simulink model "Dc_motor_pi_camp_quant"  (R2021b)
settings: Solver=VariableStepAuto  StartTime=0.0  StopTime=10.0  RelTol=1e-3
InitFcn:
  | sampling=0.01;
  | quant_err=0.0001;
settings Model: Creator=Omar  LastModifiedBy=Omar
settings DebuggingCC: UnderSpecifiedDimensionMsg=warning

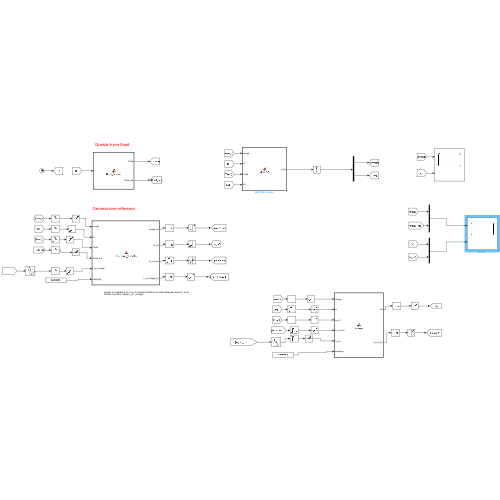
[thumbnail: Simulink's stored preview of the top-level diagram]
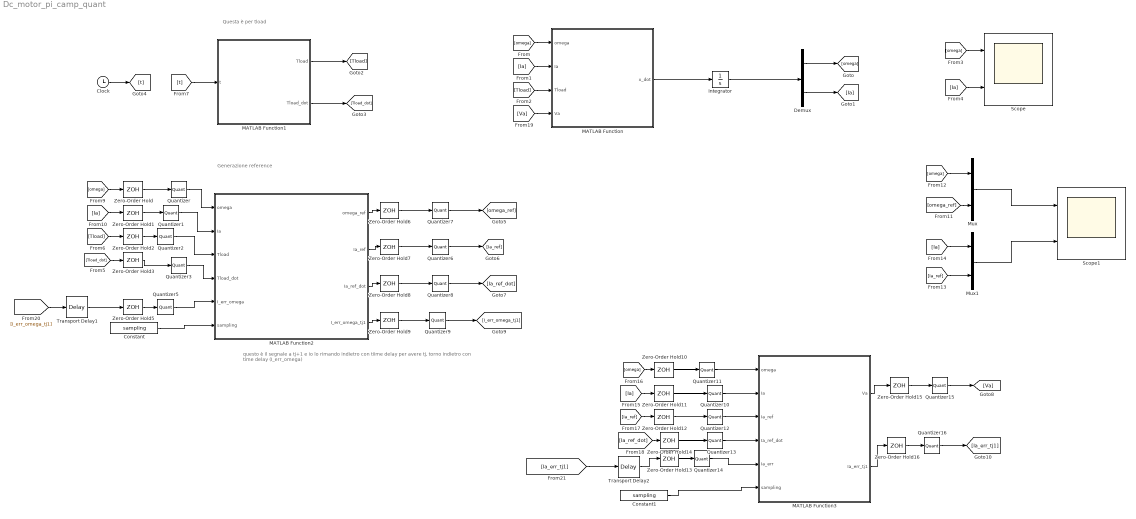
== system Dc_motor_pi_camp_quant ==
  note: questo è il segnale a tj+1 e io lo rimando indietro con tiime delay per avere tj, torno indietro con time delay (I_err_omega)
  note: Generazione reference
  note: Questa è per tload
  Clock : Clock
  Constant : Constant  Value=sampling
  Constant1 : Constant  Value=sampling
  Demux : Demux  Outputs=2
  Integrator : Integrator  InitialCondition=[0;0]
  MATLAB Function : MATLAB Function  TreatAsAtomicUnit=on
  MATLAB Function1 : MATLAB Function  TreatAsAtomicUnit=on
  MATLAB Function2 : MATLAB Function  TreatAsAtomicUnit=on
  MATLAB Function3 : MATLAB Function  TreatAsAtomicUnit=on
  Mux : Mux  Inputs=2
  Mux1 : Mux  Inputs=2
  Quantizer{,1..3,5..16} (16 alike) : Quantizer  QuantizationInterval=quant_err
  Scope : Scope  NumInputPorts=2
  Scope1 : Scope  NumInputPorts=2
  Transport Delay1 : TransportDelay  DelayTime=sampling
  Transport Delay2 : TransportDelay  DelayTime=sampling
  Zero-Order Hold{,1..3,5..16} (16 alike) : ZeroOrderHold  SampleTime=sampling
  wires:
  [t] -> MATLAB Function1/1(t)
  MATLAB Function1/2(Tload_dot) -> [Tload_dot]
  [Ia] -> MATLAB Function/2(Ia)
  MATLAB Function2/4(I_err_omega_tj1) -> Zero-Order Hold9/1
  Mux/1 -> Scope1/1
  MATLAB Function2/1(omega_ref) -> Zero-Order Hold6/1
  Clock/1 -> [t]
  MATLAB Function2/2(Ia_ref) -> Zero-Order Hold7/1
  [Ia] -> Scope/2
  [omega] -> Scope/1
  [Ia_ref] -> Zero-Order Hold12/1
  [Ia] -> Mux1/1
  [omega] -> Zero-Order Hold10/1
  [Ia_ref] -> Mux1/2
  [omega] -> Mux/1
  [Ia] -> Zero-Order Hold11/1
  Mux1/1 -> Scope1/2
  [omega_ref] -> Mux/2
  [Va] -> MATLAB Function/4(Va)
  Demux/2 -> [Ia]
  [Tload] -> MATLAB Function/3(Tload)
  Demux/1 -> [omega]
  MATLAB Function2/3(Ia_ref_dot) -> Zero-Order Hold8/1
  [omega] -> MATLAB Function/1(omega)
  MATLAB Function1/1(Tload) -> [Tload]
  MATLAB Function/1(x_dot) -> Integrator/1
  Integrator/1 -> Demux/1
  [omega] -> Zero-Order Hold/1
  Zero-Order Hold/1 -> Quantizer/1
  [Ia] -> Zero-Order Hold1/1
  Zero-Order Hold1/1 -> Quantizer1/1
  Zero-Order Hold3/1 -> Quantizer3/1
  [Tload_dot] -> Zero-Order Hold3/1
  [Tload] -> Zero-Order Hold2/1
  Zero-Order Hold2/1 -> Quantizer2/1
  [I_err_omega_tj1] -> Transport Delay1/1
  Zero-Order Hold5/1 -> Quantizer5/1
  Zero-Order Hold10/1 -> Quantizer11/1
  Zero-Order Hold11/1 -> Quantizer10/1
  Zero-Order Hold12/1 -> Quantizer12/1
  [Ia_ref_dot] -> Zero-Order Hold14/1
  [Ia_err_tj1] -> Transport Delay2/1
  MATLAB Function3/1(Va) -> Zero-Order Hold15/1
  Zero-Order Hold15/1 -> Quantizer15/1
  MATLAB Function3/2(Ia_err_tj1) -> Zero-Order Hold16/1
  Constant/1 -> MATLAB Function2/6(sampling)
  Transport Delay1/1 -> Zero-Order Hold5/1
  Constant1/1 -> MATLAB Function3/6(sampling)
  Transport Delay2/1 -> Zero-Order Hold13/1
  Zero-Order Hold13/1 -> Quantizer14/1
  Zero-Order Hold14/1 -> Quantizer13/1
  Quantizer/1 -> MATLAB Function2/1(omega)
  Quantizer1/1 -> MATLAB Function2/2(Ia)
  Quantizer2/1 -> MATLAB Function2/3(Tload)
  Quantizer3/1 -> MATLAB Function2/4(Tload_dot)
  Quantizer5/1 -> MATLAB Function2/5(I_err_omega)
  Zero-Order Hold6/1 -> Quantizer7/1
  Quantizer7/1 -> [omega_ref]
  Zero-Order Hold7/1 -> Quantizer6/1
  Quantizer6/1 -> [Ia_ref]
  Zero-Order Hold8/1 -> Quantizer8/1
  Quantizer8/1 -> [Ia_ref_dot]
  Zero-Order Hold9/1 -> Quantizer9/1
  Quantizer9/1 -> [I_err_omega_tj1]
  Quantizer11/1 -> MATLAB Function3/1(omega)
  Quantizer10/1 -> MATLAB Function3/2(Ia)
  Quantizer12/1 -> MATLAB Function3/3(Ia_ref)
  Quantizer13/1 -> MATLAB Function3/4(Ia_ref_dot)
  Quantizer14/1 -> MATLAB Function3/5(Ia_err)
  Quantizer15/1 -> [Va]
  Zero-Order Hold16/1 -> Quantizer16/1
  Quantizer16/1 -> [Ia_err_tj1]

== matlab function Dc_motor_pi_camp_quant/MATLAB Function1 ==
  data: t input; Tload output; Tload_dot output
function [Tload,Tload_dot] = Tload_function(t)
if(t<10)
    Tload=1;
else
    Tload=1.5;
end
Tload_dot=0;
end

== matlab function Dc_motor_pi_camp_quant/MATLAB Function ==
  data: omega input; x_dot output; Ia input; Tload input; Va input
function x_dot = MotorDC(omega,Ia,Tload,Va)
%definisco i parametri

k1=0.01;
k2=0.005;
J=0.01;
Bf=0.1;  % NB le variazioni parametriche influiscono moltissimo sul controllo
Ra=1;
La=0.5;

%scrivo i due modelli differenziali

omega_dot=(k1/J)*Ia-(Bf/J)*omega-(1/J)*Tload;

Ia_dot=-(Ra/La)*Ia-(k2/La)*omega+(1/La)*Va;

x_dot=[omega_dot;Ia_dot];
end

== matlab function Dc_motor_pi_camp_quant/MATLAB Function2 ==
  data: omega input; omega_ref output; Ia input; Tload input; Tload_dot input; Ia_ref output; Ia_ref_dot output; I_err_omega input; I_err_omega_tj1 output; sampling input
function [omega_ref,Ia_ref,Ia_ref_dot,I_err_omega_tj1] = Reference_generator(omega,Ia,Tload,Tload_dot,I_err_omega,sampling)
k1=0.01;
k2=0.005;
J=0.01;
Bf=0.1;
La=0.5;
kp=0.5;
kp_omega=3;  %kp legato alla velocita angolare
ki_omega=6;

%ora posso implementare le due reference
%reference omega

omega_ref=1;
omega_ref_dot=0;
omega_ref_ddot=0;
e_omega=omega-omega_ref;

%reference Ia

omega_dot=(k1/J)*Ia-(Bf/J)*omega-(1/J)*Tload;
I_err_omega_tj1= I_err_omega+sampling*(e_omega);%sarebbe integrale dell'errore al passo t(j+1) calcolata con eulero

Ia_ref=(J/k1)*(omega_ref_dot-kp_omega*(omega-omega_ref)-ki_omega*I_err_omega)+(1/k1)*(Bf*omega+Tload);
Ia_ref_dot=(J/k1)*(omega_ref_ddot-kp_omega*(omega_dot-omega_ref_dot)-ki_omega*I_err_omega_tj1)+ (1/k1)*(Bf*omega_dot+Tload_dot); %(Bf/J)*omega_dot+(1/J)*Tload_dot;
end

== matlab function Dc_motor_pi_camp_quant/MATLAB Function3 ==
  data: omega input; Va output; Ia input; Ia_ref input; Ia_ref_dot input; Ia_err input; Ia_err_tj1 output; sampling input
function [Va,Ia_err_tj1] = Controller(omega,Ia,Ia_ref,Ia_ref_dot,Ia_err,sampling)
k1=0.01;
k2=0.005;
J=0.01;
Bf=0.1;
La=0.5;
kp=0.5;
Ra=1;
kp_Ia=3; %kp del controllore legato alla corrente lo scelgo io
ki_i_Ia=6;

e_Ia=Ia-Ia_ref;
Ia_err_tj1=Ia_err+sampling*(e_Ia);

%Va=Ia*((Ra/La)*Ia+(k2/La)*omega)+Ia_ref_dot-kp_Ia*(Ia-Ia_ref);
Va=La*(Ia_ref_dot-kp_Ia*(Ia-Ia_ref)-ki_i_Ia*Ia_err_tj1)+Ra*Ia+k2*omega;
end
